simulink model "exp2"  (R2021b)
settings: Solver=VariableStepAuto  StartTime=0.0  RelTol=1e-3
libraries: slpidlib x1, simulink x1
settings Model: Creator=Lenovo  LastModifiedBy=Lenovo

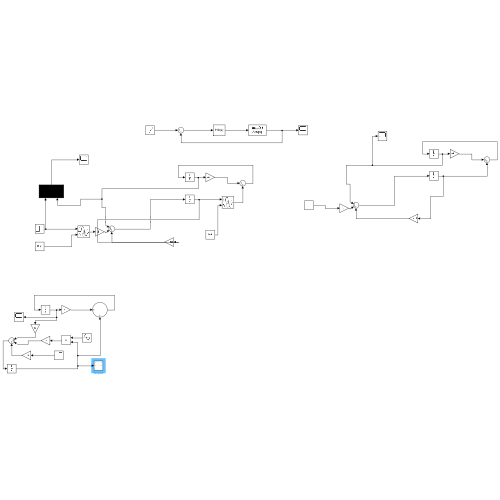
[thumbnail: Simulink's stored preview of the top-level diagram]
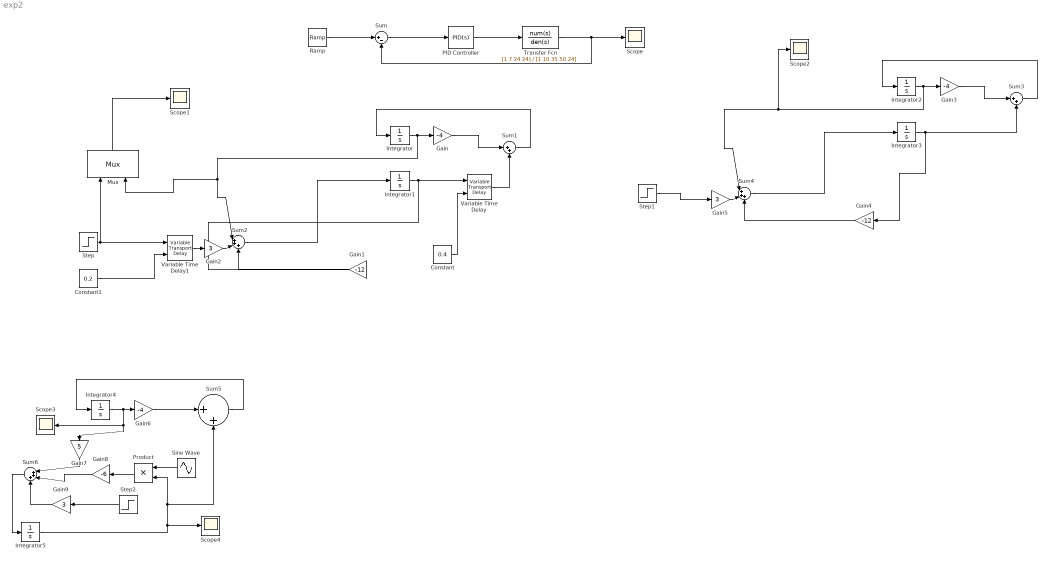
== system exp2 ==
  Constant : Constant  Value=0.4
  Constant1 : Constant  Value=0.2
  Gain : Gain  Gain=-4
  Gain1 : Gain  Gain=-12
  Gain2 : Gain  Gain=3
  Gain3 : Gain  Gain=-4
  Gain4 : Gain  Gain=-12
  Gain5 : Gain  Gain=3
  Gain6 : Gain  Gain=-4
  Gain7 : Gain  Gain=5
  Gain8 : Gain  Gain=-6
  Gain9 : Gain  Gain=3
  Integrator{,1..5} (6 alike) : Integrator
  Mux : Mux  Inputs=2
  PID Controller : slpidlib/PID Controller  Controller=PID  Form=Parallel  TimeDomain=Continuous-time  UseExternalTs=off  SampleTime=-1  IntegratorMethod=Forward Euler  FilterMethod=Forward Euler  ControllerParametersSource=internal  P=2  I=4  D=2  UseFilter=on  N=100  TunerSelectOption=Transfer Function Based (PID Tuner App)  InitialConditionSource=internal  InitialConditionForIntegrator=0  InitialConditionForFilter=0  DifferentiatorICPrevScaledInput=0  ExternalReset=none  TrackingMode=off  Kt=1  LimitOutput=off  SatLimitsSource=internal  UpperSaturationLimit=inf  LowerSaturationLimit=-inf  LinearizeAsGain=on  AntiWindupMode=none  Kb=1  POutMin=[]  POutMax=[]  IOutMin=[]  IOutMax=[]  DOutMin=[]  DOutMax=[]  NOutMin=[]  NOutMax=[]  SumOutMin=[]  SumOutMax=[]  SaturationOutMin=[]  SaturationOutMax=[]  PParamMin=[]  PParamMax=[]  IParamMin=[]  IParamMax=[]  DParamMin=[]  DParamMax=[]  NParamMin=[]  NParamMax=[]  KbParamMin=[]  KbParamMax=[]  KtParamMin=[]  KtParamMax=[]  KbOutMin=[]  KbOutMax=[]  KtOutMin=[]  KtOutMax=[]  IntegratorOutMin=[]  IntegratorOutMax=[]  FilterOutMin=[]  FilterOutMax=[]  SumI1OutMin=[]  SumI1OutMax=[]  SumI2OutMin=[]  SumI2OutMax=[]  SumI3OutMin=[]  SumI3OutMax=[]  SumI4OutMin=[]  SumI4OutMax=[]  SumDOutMin=[]  SumDOutMax=[]  DifferentiatorOutMin=[]  DifferentiatorOutMax=[]  FilterDiffOutCoefMin=[]  FilterDiffOutCoefMax=[]  ReciprocalOutMin=[]  ReciprocalOutMax=[]  SumDenOutMin=[]  SumDenOutMax=[]  SumNumOutMin=[]  SumNumOutMax=[]  DivideOutMin=[]  DivideOutMax=[]  UdiffTsProdOutMin=[]  UdiffTsProdOutMax=[]  NTsProdOutMin=[]  NTsProdOutMax=[]  UintegralTsProdOutMin=[]  UintegralTsProdOutMax=[]  UngainTsProdOutMin=[]  UngainTsProdOutMax=[]  IntegratorContinuousStateAttributes=''  IntegratorStateMustResolveToSignalObject=off  IntegratorRTWStateStorageClass=Auto  FilterContinuousStateAttributes=''  FilterStateMustResolveToSignalObject=off  FilterRTWStateStorageClass=Auto  ParallelPVariant=InternalParameters  IdealPVariant=Disabled  IVariant=InternalParameters  DVariant=InternalParameters  IntegratorVariant=Continuous  SatVariant=Disabled  AWVariant=Passthrough  PCopyVariant=Disabled  TRVariant=Disabled  FdbkBlocksVariant=Forward  IdealPFdbkVariant=Disabled  SatFdbkVariant=Disabled  DerivativeFilterVariant=ContFilter  NVariant=InternalParameters  NCopyVariant=Disabled  FilterICVariant=InternalICsFilter  IntegratorICVariant=InternalICs  ExternalResetVariant=Disabled  TRSumVariant=Passthrough  SumFdbkVariant=Disabled  SumVariant=Sum_PID  TsampFilterVariant=InternalTs  TsampNgainVariant=Passthrough  TsampIntegralVariant=Passthrough  ExternalSaturationOutDataTypeStr=Inherit: Same as second input
  Product : Product
  Ramp : simulink/Sources/Ramp  slope=1  start=0  InitialOutput=0
  Scope{,1..4} (5 alike) : Scope
  Sine Wave : Sin  SampleTime=0
  Step : Step  Time=0  SampleTime=0
  Step1 : Step  Time=0  SampleTime=0
  Step2 : Step  Time=0  SampleTime=0
  Sum : Sum  Inputs=|+-
  Sum1 : Sum  Inputs=|++
  Sum2 : Sum  Inputs=|+++
  Sum3 : Sum  Inputs=|++
  Sum4 : Sum  Inputs=|+++
  Sum5 : Sum  Inputs=|++
  Sum6 : Sum  Inputs=|+++
  Transfer Fcn : TransferFcn  Numerator=[1 7 24 24]  Denominator=[1 10 35 50 24]
  Variable Time Delay : VariableTransportDelay  VariableDelayType=Variable transport delay  MaximumDelay=0.4
  Variable Time Delay1 : VariableTransportDelay  VariableDelayType=Variable transport delay  MaximumDelay=0.2
  wires:
  Ramp/1 -> Sum/1
  Sum/1 -> PID Controller/1
  PID Controller/1 -> Transfer Fcn/1
  Transfer Fcn/1 -> Sum/2, Scope/1
  Gain1/1 -> Sum2/3
  Sum1/1 -> Integrator/1
  Step/1 -> Variable Time Delay1/1, Mux/1
  Variable Time Delay/1 -> Sum1/2
  Integrator/1 -> Mux/2, Sum2/1, Gain/1
  Integrator1/1 -> Gain1/1, Variable Time Delay/1
  Gain/1 -> Sum1/1
  Variable Time Delay1/1 -> Gain2/1
  Gain2/1 -> Sum2/2
  Sum2/1 -> Integrator1/1
  Constant/1 -> Variable Time Delay/2
  Constant1/1 -> Variable Time Delay1/2
  Integrator2/1 -> Scope2/1, Sum4/1, Gain3/1
  Sum4/1 -> Integrator3/1
  Integrator3/1 -> Sum3/2, Gain4/1
  Gain4/1 -> Sum4/3
  Gain3/1 -> Sum3/1
  Gain5/1 -> Sum4/2
  Sum3/1 -> Integrator2/1
  Step1/1 -> Gain5/1
  Gain6/1 -> Sum5/1
  Integrator5/1 -> Product/2, Sum5/2, Scope4/1
  Integrator4/1 -> Gain7/1, Scope3/1, Gain6/1
  Sum5/1 -> Integrator4/1
  Sine Wave/1 -> Product/1
  Gain7/1 -> Sum6/1
  Product/1 -> Gain8/1
  Gain8/1 -> Sum6/2
  Step2/1 -> Gain9/1
  Gain9/1 -> Sum6/3
  Sum6/1 -> Integrator5/1
  Mux/1 -> Scope1/1
